simulink model "PI_verification"  (R2021b)
settings: Solver=VariableStepAuto  StartTime=0.0  StopTime=10.0  RelTol=1e-3
values from neighbouring files (symbols this model uses):
  K = 13.45    [PI_tester.m]
  sigma = 2.2 / rise_time    (= 13.75)    [PI_tester.m]
libraries: slpidlib x1
settings Model: Creator=mluser  LastModifiedBy=mluser

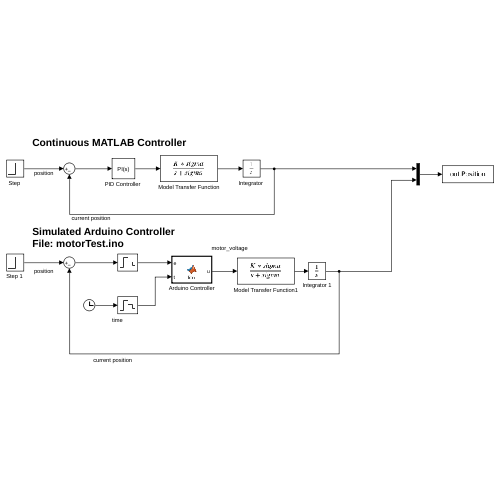
[thumbnail: Simulink's stored preview of the top-level diagram]
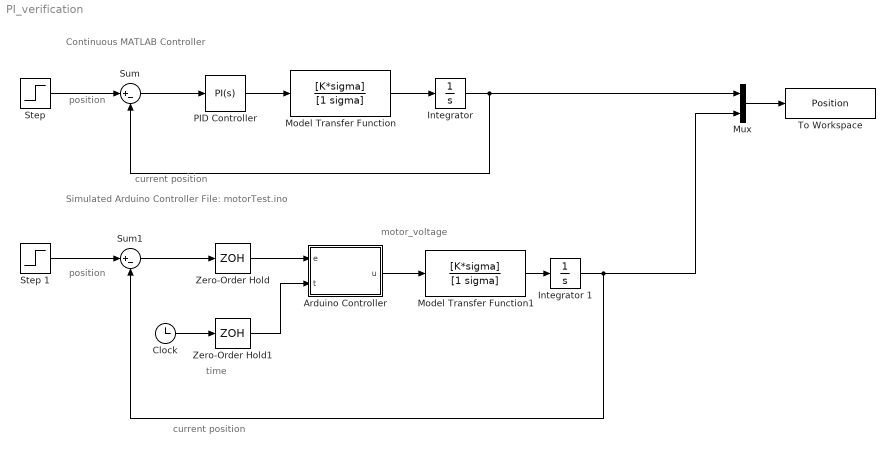
== system PI_verification ==
  note: time
  note: current position
  note: position
  note: Continuous MATLAB Controller
  note: Simulated Arduino Controller
      | File: motorTest.ino
  note: position
  note: current position
  note: motor_voltage
  Arduino Controller : MATLAB Function  TreatAsAtomicUnit=on
  Clock : Clock
  "Integrator " : Integrator
  Integrator 1 : Integrator
  Model Transfer Function : TransferFcn  Numerator=[K*sigma]  Denominator=[1 sigma]
  Model Transfer Function1 : TransferFcn  Numerator=[K*sigma]  Denominator=[1 sigma]
  Mux : Mux  Inputs=2
  "PID Controller " : slpidlib/PID Controller  Controller=PI  Form=Parallel  TimeDomain=Continuous-time  UseExternalTs=off  SampleTime=-1  IntegratorMethod=Forward Euler  FilterMethod=Forward Euler  ControllerParametersSource=internal  P=0.365942802928944  I=0.0298585215520729  D=0  UseFilter=on  N=100  TunerSelectOption=Transfer Function Based (PID Tuner App)  InitialConditionSource=internal  InitialConditionForIntegrator=0  InitialConditionForFilter=0  DifferentiatorICPrevScaledInput=0  ExternalReset=none  TrackingMode=off  Kt=1  LimitOutput=off  SatLimitsSource=internal  UpperSaturationLimit=inf  LowerSaturationLimit=-inf  LinearizeAsGain=on  AntiWindupMode=none  Kb=1  POutMin=[]  POutMax=[]  IOutMin=[]  IOutMax=[]  DOutMin=[]  DOutMax=[]  NOutMin=[]  NOutMax=[]  SumOutMin=[]  SumOutMax=[]  SaturationOutMin=[]  SaturationOutMax=[]  PParamMin=[]  PParamMax=[]  IParamMin=[]  IParamMax=[]  DParamMin=[]  DParamMax=[]  NParamMin=[]  NParamMax=[]  KbParamMin=[]  KbParamMax=[]  KtParamMin=[]  KtParamMax=[]  KbOutMin=[]  KbOutMax=[]  KtOutMin=[]  KtOutMax=[]  IntegratorOutMin=[]  IntegratorOutMax=[]  FilterOutMin=[]  FilterOutMax=[]  SumI1OutMin=[]  SumI1OutMax=[]  SumI2OutMin=[]  SumI2OutMax=[]  SumI3OutMin=[]  SumI3OutMax=[]  SumI4OutMin=[]  SumI4OutMax=[]  SumDOutMin=[]  SumDOutMax=[]  DifferentiatorOutMin=[]  DifferentiatorOutMax=[]  FilterDiffOutCoefMin=[]  FilterDiffOutCoefMax=[]  ReciprocalOutMin=[]  ReciprocalOutMax=[]  SumDenOutMin=[]  SumDenOutMax=[]  SumNumOutMin=[]  SumNumOutMax=[]  DivideOutMin=[]  DivideOutMax=[]  UdiffTsProdOutMin=[]  UdiffTsProdOutMax=[]  NTsProdOutMin=[]  NTsProdOutMax=[]  UintegralTsProdOutMin=[]  UintegralTsProdOutMax=[]  UngainTsProdOutMin=[]  UngainTsProdOutMax=[]  IntegratorContinuousStateAttributes=''  IntegratorStateMustResolveToSignalObject=off  IntegratorRTWStateStorageClass=Auto  FilterContinuousStateAttributes=''  FilterStateMustResolveToSignalObject=off  FilterRTWStateStorageClass=Auto  ParallelPVariant=InternalParameters  IdealPVariant=Disabled  IVariant=InternalParameters  DVariant=Disabled  IntegratorVariant=Continuous  SatVariant=Disabled  AWVariant=Passthrough  PCopyVariant=Disabled  TRVariant=Disabled  FdbkBlocksVariant=Forward  IdealPFdbkVariant=Disabled  SatFdbkVariant=Disabled  DerivativeFilterVariant=Disabled  NVariant=Disabled  NCopyVariant=Disabled_SignalSpec  FilterICVariant=Disabled  IntegratorICVariant=InternalICs  ExternalResetVariant=Disabled  TRSumVariant=Passthrough  SumFdbkVariant=Disabled  SumVariant=Sum_PI  TsampFilterVariant=InternalTs  TsampNgainVariant=Passthrough  TsampIntegralVariant=Passthrough  ExternalSaturationOutDataTypeStr=Inherit: Same as second input
  "Step " : Step  SampleTime=0
  "Step 1 " : Step  SampleTime=0
  Sum : Sum  Inputs=|+-
  Sum1 : Sum  Inputs=|+-
  To Workspace : ToWorkspace  VariableName=Position  SaveFormat=Timeseries  SampleTime=-1
  Zero-Order Hold : ZeroOrderHold  SampleTime=10/1000
  Zero-Order Hold1 : ZeroOrderHold  SampleTime=10/1000
  wires:
  Model Transfer Function/1 -> "Integrator "/1
  "Integrator "/1 -> Mux/1, Sum/2
  Sum/1 -> "PID Controller "/1
  "Step "/1 -> Sum/1
  "PID Controller "/1 -> Model Transfer Function/1
  "Step 1 "/1 -> Sum1/1
  Sum1/1 -> Zero-Order Hold/1
  Zero-Order Hold/1 -> Arduino Controller/1(e)
  Clock/1 -> Zero-Order Hold1/1
  Zero-Order Hold1/1 -> Arduino Controller/2(t)
  Integrator 1/1 -> Mux/2, Sum1/2
  Model Transfer Function1/1 -> Integrator 1/1
  Mux/1 -> To Workspace/1
  Arduino Controller/1(u) -> Model Transfer Function1/1

== matlab function PI_verification/Arduino Controller ==
  data: e input; u output; t input
function u = fcn(e,t)
%% Define Variables
% Control Gains
Kp = 0.36594;
Ki = 0.029859;
umax = 10;
% Memory variables
persistent I_past;
persistent t_past;
if isempty(I_past), I_past = 0; end;
if isempty(t_past), t_past = 0; end;
%% Calculate Controller output
% sample time
Ts = t - t_past;
% Integrator
I = I_past+e*Ts;
% PI control calculation
u = Kp*e+Ki*I;
% anti-windup
if abs(u)>umax
    u = sign(u)*umax;
    e = sign(e)*min(umax/Kp,abs(e));
    I = (u-Kp*e)/Ki;
end;

I_past = I;
t_past = t;
